simulink model "reichardt_array_EMD_3"  (R2018b)
settings: Solver=ode45  StartTime=0.0  StopTime=setStopTime  FixedStep=0.0005  RelTol=1e-3  EnableMultiTasking=on
model workspace (MAT data in the model file):
  bodyAmp = 0
  bodyPhase = 0
  freq = 0.832969017384
  headAmp = 0
  headPhase = 0
  imageData = [0.00228480667088 0.00685422825671 0.0114230745906 0.0159909622235 0.0205575077854 0.0251223280162 0.0296850397975 0.0342452601838 0.0388026064343 0.0433566960441 0.0479071467754 0.0524535766893 ... (8204 elements, 1x8204)]
  outputTimeList = [7.54312006335 7.61855126399 7.69398246462 7.76941366526 7.84484486589 7.92027606652 7.99570726716 8.07113846779 8.14656966842 8.22200086906 8.29743206969 8.37286327032 ... (101 elements, 1x101)]
  setStopTime = 15.0862401267
  stimAmp = 15
  temporalFilt = 0.035
  timeConstant = 0.035
libraries: visionsources x1
(part 2 of 2)

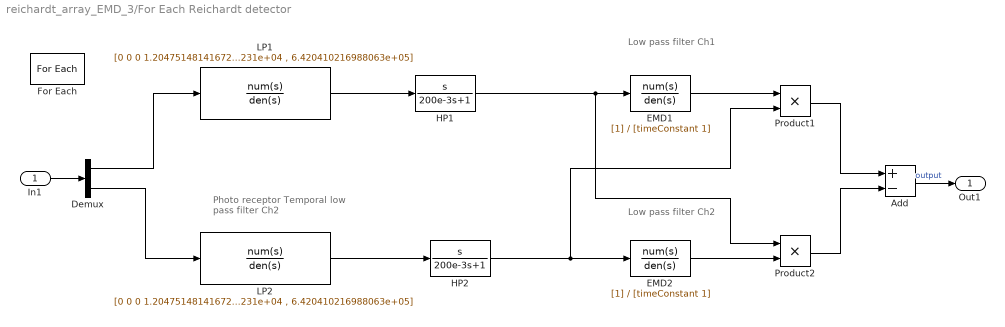
== system reichardt_array_EMD_3/For Each Reichardt detector ==
  note: Photo receptor
      | Temporal low pass filter
      | Ch2
  note: Low pass filter
      | Ch1
  note: Low pass filter
      | Ch2
  In1 : Inport  Partition=on  PartitionDimension=1  PartitionWidth=1  PartitionOffset=0
  Add : Sum  Inputs=+-
  Demux : Demux  Outputs=2
  EMD1 : TransferFcn  Denominator=[timeConstant 1]
  EMD2 : TransferFcn  Denominator=[timeConstant 1]
  For Each : ForEach  DisableCoverage=on  IndexMode=One-based
  HP1 : TransferFcn  Numerator=[1 0]  Denominator=[200e-3 1]
  HP2 : TransferFcn  Numerator=[1 0]  Denominator=[200e-3 1]
  LP1 : TransferFcn  Numerator=[0 0 0 1.204751481416720e+09]  Denominator=[1 , 2.807494939800572e+02 , 3.207046876121231e+04 , 6.420410216988063e+05]
  LP2 : TransferFcn  Numerator=[0 0 0 1.204751481416720e+09]  Denominator=[1 , 2.807494939800572e+02 , 3.207046876121231e+04 , 6.420410216988063e+05]
  Product1 : Product  RndMeth=Zero
  Product2 : Product  RndMeth=Zero
  Out1 : Outport  ConcatenationDimension=1
  wires:
  EMD1/1 -> Product1/1
  Product1/1 -> Add/1
  Product2/1 -> Add/2
  EMD2/1 -> Product2/2
  Add/1 -> Out1/1  "output"
  In1/1 -> Demux/1
  LP2/1 -> HP2/1
  LP1/1 -> HP1/1
  Demux/1 -> LP1/1
  Demux/2 -> LP2/1
  HP1/1 -> EMD1/1, Product2/1
  HP2/1 -> Product1/2, EMD2/1

== matlab function reichardt_array_EMD_3/sampleImage ==
  data: imageData input; intensity output double size=360,2; seenAngle input
function intensity = fcn(imageData,seenAngle)
%#codegen

imageWidth = length(imageData);

% Subsample with resolution of compound eye
sampleCoord = 0:359;
sampleCoord = sampleCoord + seenAngle;
sampleCoord = mod(sampleCoord,360);
temp        = interp1(linspace(0,360,imageWidth),imageData,sampleCoord);

% Create output signals
intensity = [temp(:), circshift(temp(:),-1)];
